simulink model "Decryption"  (R2024b)
settings: Solver=FixedStepAuto  StartTime=0.0  StopTime=10.0  RelTol=1e-3
undefined symbols (not defined in the file): Data_Display, descrambler, Slider
libraries: androiduilib x2, androidcommunicationlib x2, androidaudiovideolib x1, dspfdesign x1
settings Model: Creator=Tarun  LastModifiedBy=tamiz
settings OptimizationCC: EnhancedBackFolding=on  PassReuseOutputArgsThreshold=0  MaxStackSize=64  OptimizeBlockOrder=speed  DifferentSizesBufferReuse=on  OptimizationCustomize=off
settings DebuggingCC: ParameterTunabilityLossMsg=error
settings HardwareCC: ProdBitPerLong=64  ProdLargestAtomicInteger=LongLong  ProdLargestAtomicFloat=Double  ProdLongLongMode=on  ProdHWDeviceType=ARM Compatible->ARM Cortex-A (64-bit)  UseEmbeddedCoderFeatures=off  UseSimulinkCoderFeatures=off
settings SFSimCC: MATLABDynamicMemAlloc=off
settings RTWCC: Description=Embedded Coder  SystemTargetFile=ert.tlc  HardwareBoard=Android Device (64bit)  TLCOptions="-aInlineSetEventsForThisBaseRateFcn=TLC_FALSE -aSuppressMultiTaskScheduler=TLC_FALSE  -aRateBasedStepFcn=0"  TemplateMakefile=ert_default_tmf  RTWVerbose=off  Toolchain=Android SDK/NDK Tools  GPUComputeCapability=3.5
settings CodeAppCC: ForceParamTrailComments=on  OperatorAnnotations=on
settings ERTTargetCC: ERTCustomFileBanners=off  SupportContinuousTime=on  SupportNonInlinedSFcns=on  RemoveResetFunc=off  ModelStepFunctionPrototypeControlCompliant=off  InlinedParameterPlacement=Hierarchical  DynamicArrayContainerType=coder::array

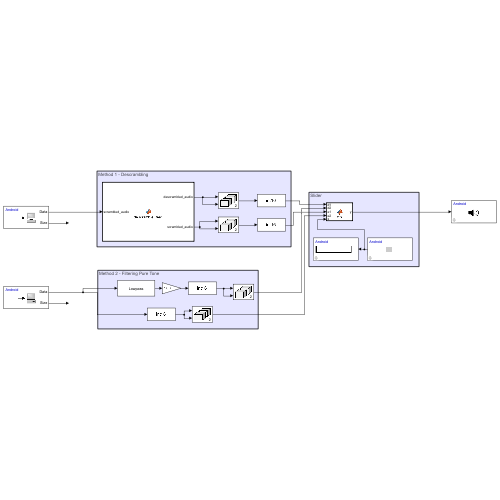
[thumbnail: Simulink's stored preview of the top-level diagram]
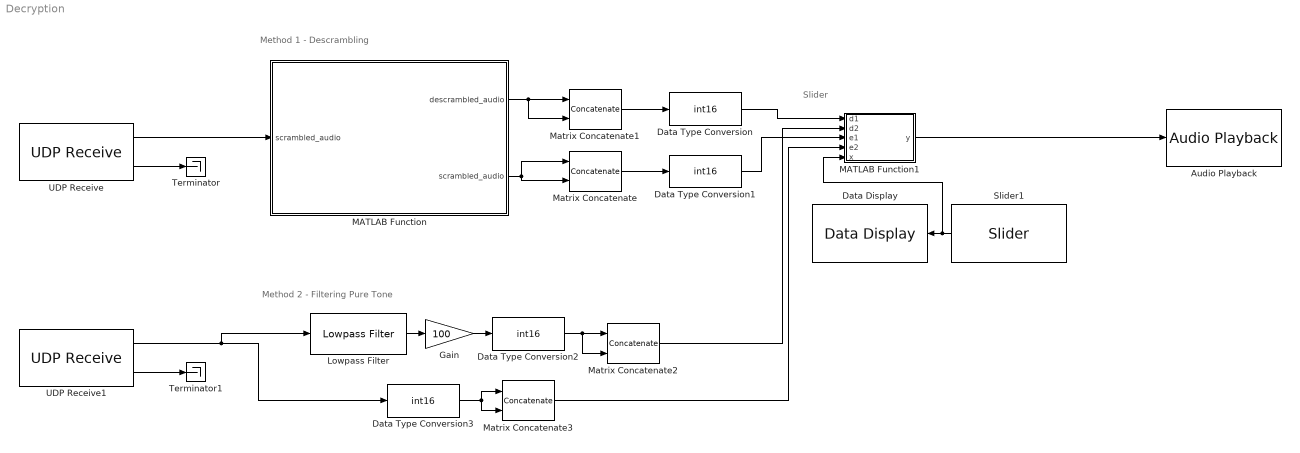
== system Decryption ==
  note: Slider
  note: Method 1 - Descrambling
  note: Method 2 - Filtering Pure Tone
  Audio Playback : androidaudiovideolib/Audio Playback  SampleFreq=44100  AudioSamplingFreq=44100  SampleTime=0.1  DeviceStr=0  QueueDuration=0  BlockPlatform=Android
  Data Display : androiduilib/Data Display  DataDisplayId=descrambler/Data_Display  Format=Float  Precision=6  SimulateUsing=Code generation  blockPlatform=Android
  Data Type Conversion{,1..3} (4 alike) : DataTypeConversion  OutDataTypeStr=int16  SaturateOnIntegerOverflow=off  RndMeth=Floor
  Gain : Gain  Gain=100
  Lowpass Filter : dspfdesign/Lowpass Filter  FilterType=FIR  DesignForMinimumOrder=on  FilterOrder=50  PassbandFrequency=6000  StopbandFrequency=8000  PassbandRipple=0.1  StopbandAttenuation=180  SampleRateMode=Specify on dialog  SampleRate=44100  SimulateUsing=Interpreted execution  roundingMode=Floor  coeffsDataTypeStr=fixdt(1,16)
  MATLAB Function : MATLAB Function  TreatAsAtomicUnit=on
  MATLAB Function1 : MATLAB Function  TreatAsAtomicUnit=on
  Matrix Concatenate{,1..3} (4 alike) : Concatenate  Mode=Multidimensional array  ConcatenateDimension=2
  Slider1 : androiduilib/Slider  Min=0  Value=0  Max=3  Resolution=1  SliderId=descrambler/Slider  SampleTime=0.05  BlockPlatform=Android
  Terminator : Terminator
  Terminator1 : Terminator
  UDP Receive : androidcommunicationlib/UDP Receive  localURL='0.0.0.0'  localPort=35000  remoteURL='0.0.0.0'  remotePort=-1  recvBufferSize=8192  signalDatatype=int16  dims=2205  isVarSize=off  showBlockingTime=off  blockingTime=0  sampletime=0.05  blockPlatform=Android
  UDP Receive1 : androidcommunicationlib/UDP Receive  localURL='0.0.0.0'  localPort=36000  remoteURL='0.0.0.0'  remotePort=-1  recvBufferSize=8192  signalDatatype=int16  dims=2205  isVarSize=off  showBlockingTime=off  blockingTime=0  sampletime=0.05  blockPlatform=Android
  wires:
  UDP Receive/2 -> Terminator/1
  UDP Receive1/2 -> Terminator1/1
  Lowpass Filter/1 -> Gain/1
  Data Type Conversion3/1 -> Matrix Concatenate3/2, Matrix Concatenate3/1
  Data Type Conversion2/1 -> Matrix Concatenate2/2, Matrix Concatenate2/1
  Gain/1 -> Data Type Conversion2/1
  UDP Receive1/1 -> Lowpass Filter/1, Data Type Conversion3/1
  UDP Receive/1 -> MATLAB Function/1("scrambled_audio ")
  MATLAB Function/1(descrambled_audio) -> Matrix Concatenate1/2, Matrix Concatenate1/1
  MATLAB Function/2(scrambled_audio) -> Matrix Concatenate/1, Matrix Concatenate/2
  Matrix Concatenate/1 -> Data Type Conversion1/1
  Matrix Concatenate1/1 -> Data Type Conversion/1
  MATLAB Function1/1(y) -> Audio Playback/1
  Data Type Conversion1/1 -> MATLAB Function1/3(e1)
  Matrix Concatenate3/1 -> MATLAB Function1/4(e2)
  Matrix Concatenate2/1 -> MATLAB Function1/2(d2)
  Slider1/1 -> MATLAB Function1/5(x), Data Display/1
  Data Type Conversion/1 -> MATLAB Function1/1(d1)

== matlab function Decryption/MATLAB Function1 ==
  data: d1 input; y output; d2 input; e1 input; e2 input; x input
function y = fcn(d1, d2, e1, e2, x)
    % Check if x equals 1
    if x == 0
        y = e1;
    elseif x==1
        y=d1;
    elseif x==2
        y=e2;
    else
        y = d2;
    end
end

== matlab function Decryption/MATLAB Function ==
  data: scrambled_audio input; descrambled_audio output; scrambled_audio output
function [descrambled_audio,scrambled_audio] = descramble_freq(scrambled_audio)
    seed=123;
    descrambled_audio = zeros(size(scrambled_audio)); 
    rng(seed, 'twister');
    n = size(scrambled_audio, 1);
    swap_indices = randperm(n);
    scrambled_audio=scrambled_audio(:,1);
    scrambled_freq_left = fft(scrambled_audio(:,1));
    [~, inverse_indices] = sort(swap_indices);
    descrambled_freq_left = scrambled_freq_left(inverse_indices);
    descrambled_audio(:,1) = real(ifft(descrambled_freq_left));
end
